simulink model "TVC_AIR_RESISTANCE"  (R2025b)
settings: Solver=VariableStepAuto  StartTime=0.0  StopTime=10  RelTol=1e-3
libraries: simulink_extras x2, dspsrcs4 x1, aerolibasang x1
settings Model: Creator=Gurjinder  LastModifiedBy=Gurjinder

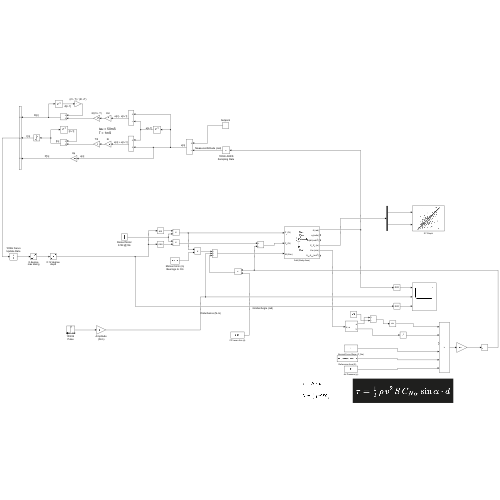
[thumbnail: Simulink's stored preview of the top-level diagram]
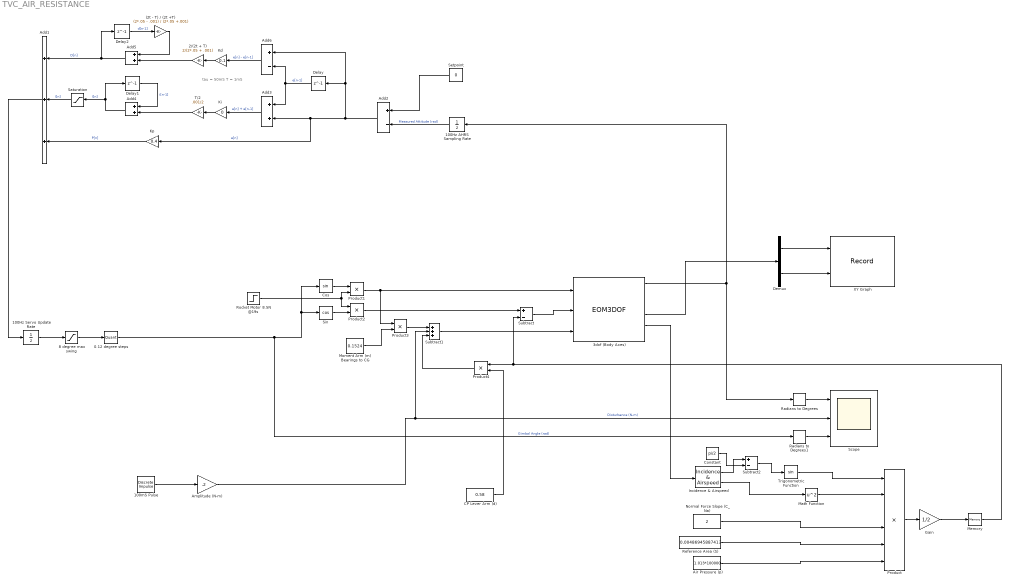
== system TVC_AIR_RESISTANCE ==
  note: tau = 50mS
      | T = 1mS
  (2t - T) / (2t +T) : Gain  Gain=(2*.05 - .001) / (2*.05 +.001)
  0.12 degree steps : Quantizer  QuantizationInterval=0.0021
  100Hz AHRS Sampling Rate : UnitDelay  SampleTime=.01  HasFrameUpgradeWarning=on
  100Hz Servo Update Rate : UnitDelay  SampleTime=.01  HasFrameUpgradeWarning=on
  100mS Pulse : dspsrcs4/Discrete  Impulse  SFcnStateName=COUNT  Delay=10  SampleTime=.1  FrameSample=1  OutputFrames=off  dataType=double  isSigned=on  wordLen=16  udDataType=sfix(16)  fracBitsMode=Best precision  numFracBits=15  OutDataTypeStr=double  LastOutDataTypeStr=double
      settings: SFcnIsStateOwnerBlock=on
  2/(2t + T) : Gain  Gain=2/(2*.05 + .001)
  3dof (Body Axes) : EOM3DOF  v_ini=0.000001  mass=0.618  Iyy=0.033  g=-9.81
  8 degree max swing : Saturate  UpperLimit=0.14  LowerLimit=-0.14
  Add1 : Sum  Inputs=+++
  Add2 : Sum  Inputs=+-
  Add3 : Sum
  Add4 : Sum
  Add5 : Sum
  Add6 : Sum  Inputs=+-
  Air Pressure (p) : Constant  Value=1.013*100000
  Amplitude (N-m) : Gain  Gain=.2
  CP Lever Arm (d) : Constant  Value=0.58
  Constant : Constant  Value=pi/2
  Cos : Trigonometry
  Delay : Delay  DelayLength=1  InitialCondition=0  SampleTime=.001
  Delay1 : Delay  DelayLength=1  InitialCondition=0  SampleTime=.001
  Delay2 : Delay  DelayLength=1  InitialCondition=0  SampleTime=.001
  Demux : Demux  Outputs=2
  Gain : Gain  Gain=1/2
  Incidence & Airspeed : aerolibasang/Incidence  & Airspeed
  Kd : Gain  Gain=0.1
  Ki : Gain  Gain=0
  Kp : Gain  Gain=0.4
  Math Function : Math  Operator=square
  Memory : Memory
  Moment Arm (m) Bearings to CG : Constant  Value=0.1524
  Normal Force Slope (C_Na) : Constant  Value=2
  Product : Product  Inputs=6
  Product{1..4} (4 alike) : Product
  Radians to Degrees : simulink_extras/Transformations/Radians to Degrees
  Radians to Degrees1 : simulink_extras/Transformations/Radians to Degrees
  Reference Area (S) : Constant  Value=0.00486945887413
  Rocket Motor 8.5N @19s : Step  Time=19  Before=8.5  After=0  SampleTime=0
  Saturation : Saturate  UpperLimit=3  LowerLimit=-3
  Scope : Scope  NumInputPorts=3
      settings: ActiveDisplayYMinimum=-5.7020658962803186  ActiveDisplayYMaximum=6.7997723848579055
  Setpoint : Constant  Value=0
  Sin : Trigonometry  Operator=cos
  Subtract : Sum  Inputs=+-
  Subtract1 : Sum  Inputs=+++
  Subtract2 : Sum  Inputs=+-
  T/2 : Gain  Gain=.001/2
  Trigonometric Function : Trigonometry
  XY Graph : Record  NumPorts=2.0  FileSettingsInternal="{\"entries\":[{\"content\":{\"excelSettings\":{\"content\":{},\"type\":\"Streamout.ExcelSettings\"},\"parquetSettings\":{\"content\":{},\"type\":\"Streamout.ParquetSettings\"}},\"type\":\"Streamout.FileSettingStorage\",\"uuid\":\"\"}],\"packageUris\":[\"http:\\/\\/schema.mathworks.com\\/mf0\\/streamout_blocks\\/R2020a\"],\"version\":\"1.0\"}"  FrameSettings=[0, 0]  Layout=[1 1]  SignalsInternal="{\"entries\":[{\"content\":{\"signals\":[{\"content\":{\"blockPath\":[],\"dimensions\":[1],\"domain\":\"\",\"lineColor\":\"#a2142f\",\"plots\":[ 1 ],\"port\":1,\"sid\":[\"\"],\"signalID\":1,\"signalName\":\"Demux:1\"},\"type\":\"RecordBlkView.Signal\",\"uuid\":\"\"},{\"content\":{\"blockPath\":[],\"dimensions\":[1],\"domain\":\"\",\"lineColor\":\"#139fff\",\"plots\":[ 1 ],\"port\":2,\"sid\":[\"\"],\"signalID\":2,\"signalName\":\"Demux:2\"},\"type\":\"RecordBlkView.Signal\",\"uuid\":\"\"}]},\"type\":\"RecordBlkView.InputSignals\",\"uuid\":\"\"}],\"packageUris\":[\"http:\\/\\/schema.mathworks.com\\/mf0\\/streamout_blocks\\/R2020a\"],\"version\":\"1.0\"}"  VisualizationBindings="{\"xyplotplugin\":{\"info\":[{\"series\":[{\"bindingParametersList\":[{\"parameter\":\"X-Axis\",\"signalID\":1,\"signalName\":\"Demux:1\"},{\"parameter\":\"Y-Axis\",\"signalID\":2,\"signalName\":\"Demux:2\"}],\"seriesID\":0}],\"subplotID\":1}]}}"  CompatibilityTag=XY
  wires:
  Cos/1 -> Product1/1
  8 degree max swing/1 -> 0.12 degree steps/1
  0.12 degree steps/1 -> Radians to Degrees1/1, Cos/1, Sin/1  "Gimbal Angle (rad)"
  100Hz Servo Update Rate/1 -> 8 degree max swing/1
  Sin/1 -> Product2/2
  Rocket Motor 8.5N @19s/1 -> Product2/1, Product1/2
  100mS Pulse/1 -> Amplitude (N-m)/1
  Subtract1/1 -> 3dof (Body Axes)/3
  Amplitude (N-m)/1 -> Scope/2, Subtract1/2  "Disturbance (N-m)"
  Product1/1 -> 3dof (Body Axes)/1, Product3/1
  Moment Arm (m) Bearings to CG/1 -> Product3/2
  Product3/1 -> Subtract1/1
  Ki/1 -> T/2/1
  2/(2t + T)/1 -> Add5/2
  Setpoint/1 -> Add2/1
  Kp/1 -> Add1/3  "P[n]"
  Delay1/1 -> Add4/1  "i[n-1]"
  Delay2/1 -> (2t - T) / (2t +T)/1  "d[n-1]"
  T/2/1 -> Add4/2
  Kd/1 -> 2/(2t + T)/1
  Add3/1 -> Ki/1  "e[n] + e[n-1]"
  Add4/1 -> Saturation/1, Delay1/1  "I[n]"
  100Hz AHRS Sampling Rate/1 -> Add2/2  "Measured Attitude (rad)"
  Add6/1 -> Kd/1  "e[n] - e[n-1]"
  Saturation/1 -> Add1/2  "I[n]"
  Add2/1 -> Add3/2, Kp/1, Delay/1, Add6/1  "e[n]"
  Add5/1 -> Add1/1, Delay2/1  "D[n]"
  Delay/1 -> Add3/1, Add6/2  "e[n-1]"
  (2t - T) / (2t +T)/1 -> Add5/1
  Add1/1 -> 100Hz Servo Update Rate/1
  3dof (Body Axes)/1 -> 100Hz AHRS Sampling Rate/1, Radians to Degrees/1
  Radians to Degrees/1 -> Scope/1
  Radians to Degrees1/1 -> Scope/3
  3dof (Body Axes)/4 -> Demux/1
  Demux/1 -> XY Graph/1
  Demux/2 -> XY Graph/2
  3dof (Body Axes)/5 -> Incidence & Airspeed/1
  Product/1 -> Gain/1
  Normal Force Slope (C_Na)/1 -> Product/4
  Reference Area (S)/1 -> Product/5
  Air Pressure (p)/1 -> Product/6
  Trigonometric Function/1 -> Product/1
  Math Function/1 -> Product/2
  Incidence & Airspeed/2 -> Math Function/1
  CP Lever Arm (d)/1 -> Product4/2
  Product4/1 -> Subtract1/3
  Product2/1 -> Subtract/1
  Subtract/1 -> 3dof (Body Axes)/2
  Incidence & Airspeed/1 -> Subtract2/1
  Constant/1 -> Subtract2/2
  Subtract2/1 -> Trigonometric Function/1
  Gain/1 -> Memory/1
  Memory/1 -> Subtract/2, Product4/1
